simulink model "contDenAutoTuningbutton"  (R2021b)
settings: Solver=ode3  StartTime=0.0  StopTime=2500  FixedStep=0.2  RelTol=1e-3  EnableMultiTasking=on
undefined symbols (not defined in the file or in its folder): buttonSim, disturbanceSim, relayBut, setSimA, tuningfunc
settings Model: Creator=issme  LastModifiedBy=ismt
settings SolverCC: AlgebraicLoopSolver=TrustRegion
settings DataIOCC: SaveFormat=Array  SignalLoggingSaveFormat=ModelDataLogs  ReturnWorkspaceOutputs=off  OutputSaveName=yout_Autotune
settings OptimizationCC: ExpressionDepthLimit=2147483647  InitFltsAndDblsToZero=on  LifeSpan=inf
settings DebuggingCC: UnderspecifiedInitializationDetection=Classic  MergeDetectMultiDrivingBlocksExec=none  SolverPrmCheckMsg=warning  FcnCallInpInsideContextMsg=warning  StateNameClashWarn=warning  SFUnexpectedBacktrackingDiag=warning  SFNoUnconditionalDefaultTransitionDiag=warning  SFExecutionAtInitializationDiag=none  SFMachineParentedDataDiag=warning  ArithmeticOperatorsInVariantConditions=warning
settings HardwareCC: ProdBitPerPointer=32  ProdBitPerSizeT=32  ProdBitPerPtrDiffT=32  ProdLargestAtomicFloat=None  ProdIntDivRoundTo=Undefined  ProdEndianess=Unspecified  ProdWordSize=32  ProdHWDeviceType=32-bit Generic
settings ModelReferenceCC: PropagateSignalLabelsOutOfModel=off
settings CodeAppCC: StateflowObjectComments=on
settings GRTTargetCC: TargetLangStandard=C89/C90 (ANSI)  CombineOutputUpdateFcns=off  GRTInterface=on
settings ConfigComp: CovMetricSettings=dw  CovSaveCumulativeToWorkspaceVar=on  CovSaveSingleToWorkspaceVar=on

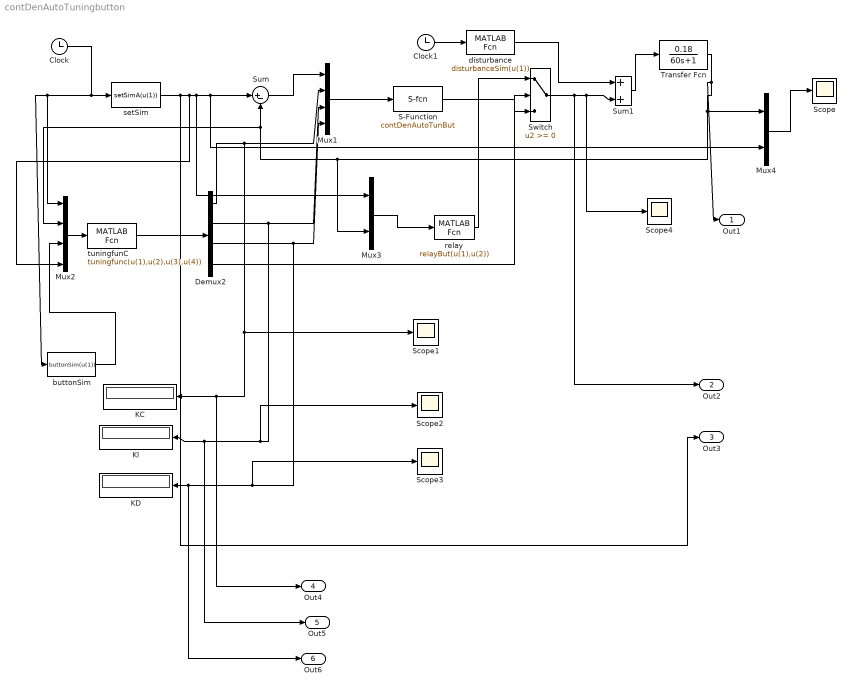
== system contDenAutoTuningbutton ==
  Clock : Clock
  Clock1 : Clock
  Demux2 : Demux
  KC : Display
  KD : Display
  KI : Display
  Mux1 : Mux
  Mux2 : Mux
  Mux3 : Mux  Inputs=2
  Mux4 : Mux  Inputs=2
  S-Function : S-Function  FunctionName=contDenAutoTunBut  SFunctionDeploymentMode=off  EnableBusSupport=off
  Scope{,1..4} (5 alike) : Scope
  Sum : Sum  Inputs=|+-
  Sum1 : Sum  Inputs=|++
  Switch : Switch  SampleTime=0.2
  Transfer Fcn : TransferFcn  Numerator=[0.18]  Denominator=[60 1]
  buttonSim : MATLABFcn  MATLABFcn=buttonSim(u(1))  OutputDimensions=1  SampleTime=0.2
  disturbance : MATLABFcn  MATLABFcn=disturbanceSim(u(1))  OutputDimensions=1  SampleTime=0.2
  relay : MATLABFcn  MATLABFcn=relayBut(u(1),u(2))  OutputDimensions=1  SampleTime=0.2
  setSim : MATLABFcn  MATLABFcn=setSimA(u(1))  OutputDimensions=1  SampleTime=0.2
  tuningfunC : MATLABFcn  MATLABFcn=tuningfunc(u(1),u(2),u(3),u(4))  OutputDimensions=4  SampleTime=0.2
  Out1 : Outport
  Out2 : Outport  Port=2
  Out3 : Outport  Port=3
  Out4 : Outport  Port=4
  Out5 : Outport  Port=5
  Out6 : Outport  Port=6
  wires:
  setSim/1 -> Mux2/4, Mux4/2, Sum/1, Mux3/1, Out3/1
  Transfer Fcn/1 -> Sum/2, Mux2/2, Mux3/2, Mux4/1, Out1/1
  relay/1 -> Switch/1
  Sum/1 -> Mux1/1
  Mux1/1 -> S-Function/1
  Clock/1 -> setSim/1, Mux2/1, buttonSim/1
  tuningfunC/1 -> Demux2/1
  Demux2/1 -> Mux1/2, KC/1, Out4/1, Scope1/1
  Demux2/2 -> Mux1/3, Scope2/1, KI/1, Out5/1
  Demux2/3 -> Mux1/4, Scope3/1, KD/1, Out6/1
  Demux2/4 -> Switch/2
  buttonSim/1 -> Mux2/3
  Mux2/1 -> tuningfunC/1
  S-Function/1 -> Switch/3
  Mux3/1 -> relay/1
  Clock1/1 -> disturbance/1
  Sum1/1 -> Transfer Fcn/1
  Switch/1 -> Out2/1, Scope4/1, Sum1/2
  disturbance/1 -> Sum1/1
  Mux4/1 -> Scope/1
